simulink model "Color_recog_drone"  (R2023b)
settings: Solver=FixedStepAuto  StartTime=0.0  StopTime=inf  RelTol=1e-3  EnableMultiTasking=on
InitFcn:
  | load('BusDefinitions.mat')
  | codertarget.parrot.internal.checkImageBlocks(gcs)
undefined symbols (not defined in the file): codertarget, gray, Ts
libraries: matrix_library x3, simulink x1, parrotlib x1
settings Model: SimulationMode=external  ExtModeTrigDuration=80  Creator=Thaarun  LastModifiedBy=Thaarun
settings SolverCC: AlgebraicLoopSolver=TrustRegion  PositivePriorityOrder=on
settings OptimizationCC: ReuseModelBlockBuffer=off  PassReuseOutputArgsThreshold=0  MaxStackSize=64
settings DebuggingCC: ParameterTunabilityLossMsg=error  UnconnectedInputMsg=warning  UnconnectedOutputMsg=warning  UnconnectedLineMsg=warning  ArithmeticOperatorsInVariantConditions=warning
settings HardwareCC: ProdBitPerPointer=32  ProdBitPerSizeT=32  ProdBitPerPtrDiffT=32  ProdLargestAtomicInteger=Long  ProdWordSize=32  ProdHWDeviceType=ARM Compatible->ARM 9  UseEmbeddedCoderFeatures=off  UseSimulinkCoderFeatures=off
settings ModelReferenceCC: EnableRefExpFcnMdlSchedulingChecks=on
settings SFSimCC: SimUseLocalCustomCode=off  MATLABDynamicMemAlloc=off
settings RTWCC: Description=Embedded Coder  SystemTargetFile=ert.tlc  HardwareBoard=PARROT Mambo  TemplateMakefile=ert_default_tmf  RTWVerbose=off  RTWUseLocalCustomCode=off  Toolchain=Sourcery G++ Lite GNU Toolchain for Drones  DLArmComputeVersion=19.05
settings CodeAppCC: ForceParamTrailComments=on  OperatorAnnotations=on  MangleLength=10  StateflowObjectComments=on
settings ERTTargetCC: ERTCustomFileBanners=off  SupportContinuousTime=on  SupportNonInlinedSFcns=on  RemoveResetFunc=off  ModelStepFunctionPrototypeControlCompliant=off  ExtMode=on  ExtModeMaxTrigDuration=80  ExtModeMexArgs='192.168.3.1' 1 17725  ERTSrcFileBannerTemplate=codertarget_code_template.cgt  ERTHdrFileBannerTemplate=codertarget_code_template.cgt  ERTDataSrcFileTemplate=codertarget_code_template.cgt  ERTDataHdrFileTemplate=codertarget_code_template.cgt

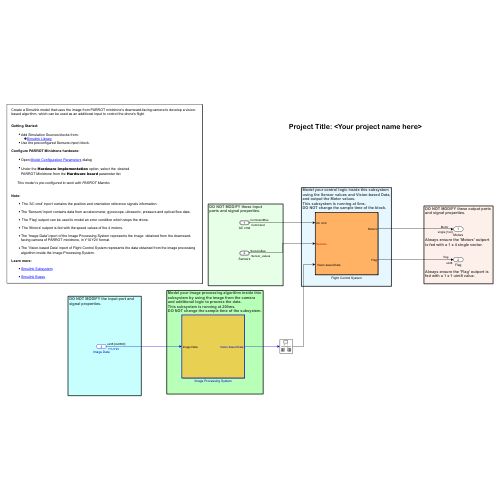
[thumbnail: Simulink's stored preview of the top-level diagram]
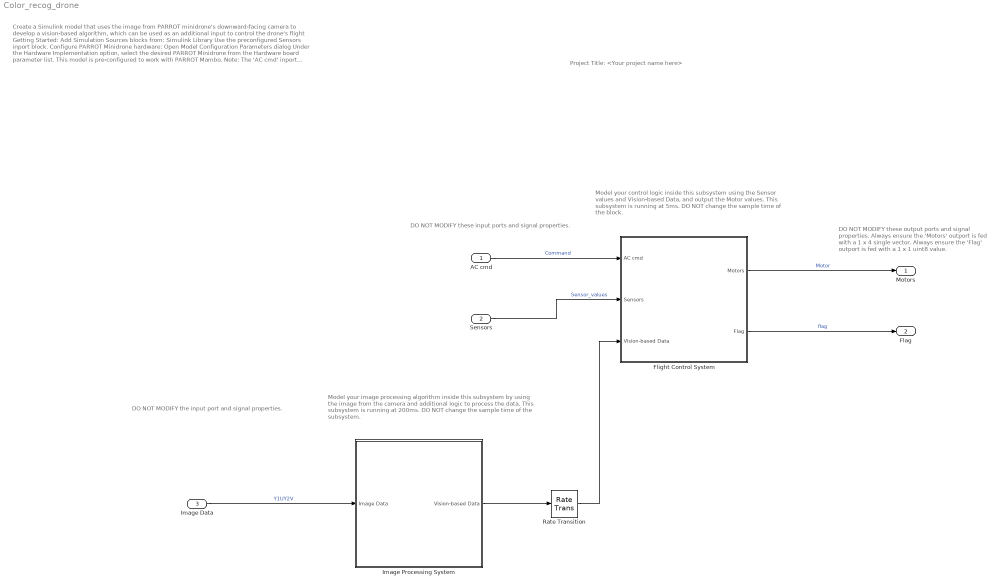
== system Color_recog_drone ==
  note: Model your control logic inside this subsystem
      | using the Sensor values and Vision-based Data,
      | and output the Motor values.
      | This subsystem is running at 5ms.
      | DO NOT change the sample time of the block.
  note: DO NOT MODIFY these output ports
      | and signal properties.
      |
      |
      |
      |
      |
      | Always ensure the 'Motors' outport
      | is fed with a 1 x 4 single vector.
      |
      |
      |
      |
      |
      | Always ensure the 'Flag' outport is
      | fed with a 1 x 1 uint8 value.
  note: DO NOT MODIFY these input
      | ports and signal properties.
  note: Create a Simulink model that uses the image from PARROT minidrone's downward-facing camera to develop a vision-based algorithm, which can be used as an additional input to control the drone's flight
      |
      | Getting Started:
      |
      | Add Simulation Sources blocks from:
      | Simulink Library
      | Use the preconfigured Sensors inport block.
      |
      | Configure PARROT Minidrone hardware:
      |
      | Open Model Configuration Parameters dialog
      |
      | Under the Hardware Implementation option, select the desired
      | PARROT Minidrone from the Hardware board parameter list.
      |
      | This model is pre-configured to work with PARROT Mambo.
      |
      | Note:
      |
      | The 'AC cmd' inport contains the position and orientation reference signals information.
      | The 'Sensors' inport contains data from accelerometer, gyroscope, ultrasonic, pressure and optical flow data.
      | The 'Flag' outport can be used to model an error condition which stops the drone.
      | The 'Motors' outport is fed with the speed values of the 4 motors.
      | The 'Image Data' inport of the Image Processing System represents the image obtained from the downward-facing camera of PARROT minidrone, in Y1UY2V format.
      | The 'Vision-based Data' inport of Flight Control System represents the data obtained from the image processing algorithm inside the Image Processing System.
      | Learn more:
      |
      | Simulink Subsystem
      | Simulink Buses
  note: Project Title: <Your project name here>
  note: DO NOT MODIFY the input port and
      | signal properties.
  note: Model your image processing algorithm inside this
      | subsystem by using the image from the camera
      | and additional logic to process the data.
      | This subsystem is running at 200ms.
      | DO NOT change the sample time of the subsystem.
  AC cmd : Inport  OutDataTypeStr=Bus: CommandBus  BusOutputAsStruct=on
  Sensors : Inport  Port=2  OutDataTypeStr=Bus: SensorsBus  BusOutputAsStruct=on
  Image Data : Inport  Tag=IP_IN  InitFcn=codertarget.parrot.internal.inportCallback(gcb);  Port=3  OutDataTypeStr=uint8  PortDimensions=[4 9600]  BusOutputAsStruct=on
  Flight Control System : Subsystem  InitFcn=codertarget.parrot.internal.fcsSubsystemCallback(gcb);  TreatAsAtomicUnit=on  SystemSampleTime=Ts
  Image Processing System : Subsystem  Tag=IP_SUB  InitFcn=codertarget.parrot.internal.ipSubsystemCallback(gcb);  TreatAsAtomicUnit=on  SystemSampleTime=40*Ts  RTWFcnName=ImageFunction
      settings: RTWSystemCode=Inline  RTWFcnNameOpts=User specified
  Rate Transition : RateTransition  Deterministic=off
  Motors : Outport  OutDataTypeStr=single  PortDimensions=[1 4]  VectorParamsAs1DForOutWhenUnconnected=off
  Flag : Outport  Port=2  OutDataTypeStr=uint8  PortDimensions=1  VectorParamsAs1DForOutWhenUnconnected=off
  wires:
  Flight Control System/1(Motors) -> Motors/1  "Motor"
  AC cmd/1 -> Flight Control System/1(AC cmd)  "Command"
  Sensors/1 -> Flight Control System/2(Sensors)  "Sensor_values"
  Flight Control System/2(Flag) -> Flag/1  "flag"
  Image Data/1 -> Image Processing System/1(Image Data)  "Y1UY2V"
  Rate Transition/1 -> Flight Control System/3(" Vision-based Data")
  Image Processing System/1(" Vision-based Data") -> Rate Transition/1

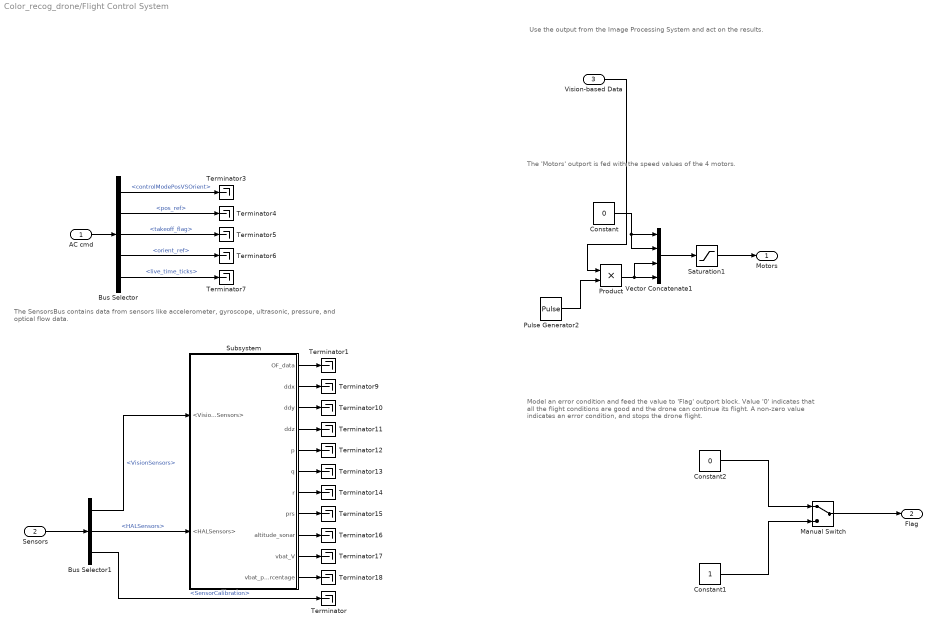
== system Color_recog_drone/Flight Control System ==
  note: The 'Motors' outport is fed with the speed values of the 4 motors.
  note: Model an error condition and feed the value to 'Flag' outport block.
      | Value '0' indicates that all the flight conditions are good and the drone
      | can continue its flight.
      | A non-zero value indicates an error condition, and stops the drone
      | flight.
  note: The SensorsBus contains data from sensors like
      | accelerometer, gyroscope, ultrasonic, pressure,
      | and optical flow data.
  note: Use the output from the Image Processing System and act on the
      | results.
  AC cmd : Inport
  Sensors : Inport  Port=2
  " Vision-based Data" : Inport  Port=3
  Bus Selector : BusSelector  OutputSignals=controlModePosVSOrient,pos_ref,takeoff_flag,orient_ref,live_time_ticks
  Bus Selector1 : BusSelector  OutputSignals=VisionSensors,HALSensors,SensorCalibration
  Constant : Constant  Value=0
  Constant1 : Constant  OutDataTypeStr=uint8
  Constant2 : Constant  Value=0  OutDataTypeStr=uint8
  Manual Switch : ManualSwitch
  Product : Product
  Pulse Generator2 : DiscretePulseGenerator  Amplitude=400  Period=800  PulseWidth=400  PhaseDelay=400  SampleTime=Ts
  Saturation1 : Saturate  UpperLimit=500  LowerLimit=0  OutDataTypeStr=single
  Subsystem : Subsystem
  Terminator{,1,3..7,9..18} (17 alike) : Terminator
  Vector Concatenate1 : Concatenate  NumInputs=4
  Motors : Outport  VectorParamsAs1DForOutWhenUnconnected=off
  Flag : Outport  Port=2  VectorParamsAs1DForOutWhenUnconnected=off
  wires:
  AC cmd/1 -> Bus Selector/1
  Sensors/1 -> Bus Selector1/1
  Bus Selector/1 -> Terminator3/1  "<controlModePosVSOrient>"
  Bus Selector/2 -> Terminator4/1  "<pos_ref>"
  Bus Selector/3 -> Terminator5/1  "<takeoff_flag>"
  Bus Selector/4 -> Terminator6/1  "<orient_ref>"
  Bus Selector/5 -> Terminator7/1  "<live_time_ticks>"
  Manual Switch/1 -> Flag/1
  Constant2/1 -> Manual Switch/1
  Constant1/1 -> Manual Switch/2
  Vector Concatenate1/1 -> Saturation1/1
  Pulse Generator2/1 -> Product/2
  Saturation1/1 -> Motors/1
  Bus Selector1/1 -> Subsystem/1(<VisionSensors>)  "<VisionSensors>"
  Bus Selector1/2 -> Subsystem/2(<HALSensors>)  "<HALSensors>"
  Bus Selector1/3 -> Terminator/1  "<SensorCalibration>"
  Subsystem/1(OF_data) -> Terminator1/1
  Subsystem/2(ddx) -> Terminator9/1
  Subsystem/3(ddy) -> Terminator10/1
  Subsystem/4(ddz) -> Terminator11/1
  Subsystem/5(p) -> Terminator12/1
  Subsystem/7(r) -> Terminator14/1
  Subsystem/8(prs) -> Terminator15/1
  Subsystem/9(altitude_sonar) -> Terminator16/1
  Subsystem/10(vbat_V) -> Terminator17/1
  Subsystem/11(vbat_percentage) -> Terminator18/1
  Subsystem/6(q) -> Terminator13/1
  Constant/1 -> Vector Concatenate1/2, Vector Concatenate1/1
  " Vision-based Data"/1 -> Product/1
  Product/1 -> Vector Concatenate1/3, Vector Concatenate1/4

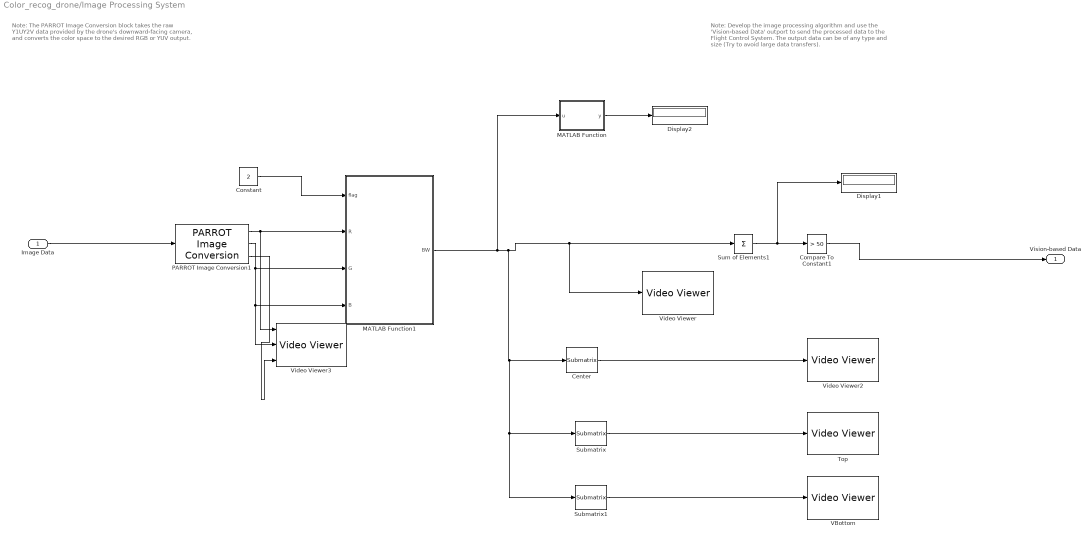
== system Color_recog_drone/Image Processing System ==
  note: Note:
      |
      | Develop the image processing algorithm and use the 'Vision-based Data' outport to send the processed data to the Flight Control System. The output data can be of any type and size (Try to avoid large data transfers).
  note: Note:
      |
      | The PARROT Image Conversion block takes the raw Y1UY2V data provided by the drone's downward-facing camera, and converts the color space to the desired RGB or YUV output.
  Image Data : Inport
  Center : matrix_library/Submatrix  RowSpan=Range of rows  RowStartMode=Offset from middle  RowStartIndex=-10  RowEndMode=Offset from middle  RowEndIndex=10  ColSpan=Range of columns  ColStartMode=Offset from middle  ColStartIndex=-10  ColEndMode=Offset from middle  ColEndIndex=10
  Compare To Constant1 : simulink/Logic and Bit Operations/Compare To Constant  relop=>  const=50  OutDataTypeStr=boolean
  Constant : Constant  Value=2  OutDataTypeStr=int8
  Display1 : Display
  Display2 : Display
  MATLAB Function : MATLAB Function  TreatAsAtomicUnit=on
  MATLAB Function1 : MATLAB Function  TreatAsAtomicUnit=on
  PARROT Image Conversion1 : parrotlib/PARROT Image Conversion  Tag=IP_FORMAT  ImageFormat=RGB  R=on  Y=on  G=on  U=on  B=on  V=on
  Submatrix : matrix_library/Submatrix  RowSpan=Range of rows  RowStartMode=First  RowStartIndex=10  RowEndMode=Index  RowEndIndex=30  ColSpan=Range of columns  ColStartMode=First  ColStartIndex=-10  ColEndMode=Last  ColEndIndex=10
  Submatrix1 : matrix_library/Submatrix  RowSpan=Range of rows  RowStartMode=Index  RowStartIndex=90  RowEndMode=Last  RowEndIndex=30  ColSpan=Range of columns  ColStartMode=First  ColStartIndex=-10  ColEndMode=Last  ColEndIndex=10
  Sum of Elements1 : Sum  Inputs=+  OutDataTypeStr=uint16
  Top : VideoViewer  colormapValue=gray(256)  FigPos=[957 1001.2 417.6 304]
  VBottom : VideoViewer  colormapValue=gray(256)  FigPos=[29.8 702 417.6 304]
  Video Viewer : VideoViewer  colormapValue=gray(256)  FigPos=[969 641.2 424.8 352.8]
  Video Viewer2 : VideoViewer  colormapValue=gray(256)  FigPos=[1096.2 1246.8 567.2 484]
  Video Viewer3 : VideoViewer  imagePorts=separate color signals  colormapValue=gray(256)  FigPos=[122.6 846.8 766.4 672]
  " Vision-based Data" : Outport  VectorParamsAs1DForOutWhenUnconnected=off
  wires:
  PARROT Image Conversion1/1 -> Video Viewer3/1, MATLAB Function1/2(R)
  MATLAB Function1/1(BW) -> MATLAB Function/1(u), Submatrix1/1, Submatrix/1, Center/1, Video Viewer/1, Sum of Elements1/1
  PARROT Image Conversion1/2 -> Video Viewer3/2, MATLAB Function1/4(B), MATLAB Function1/3(G)
  Sum of Elements1/1 -> Display1/1, Compare To Constant1/1
  Image Data/1 -> PARROT Image Conversion1/1
  PARROT Image Conversion1/3 -> Video Viewer3/3
  Compare To Constant1/1 -> " Vision-based Data"/1
  MATLAB Function/1(y) -> Display2/1
  Center/1 -> Video Viewer2/1
  Submatrix/1 -> Top/1
  Submatrix1/1 -> VBottom/1
  Constant/1 -> MATLAB Function1/1(flag)

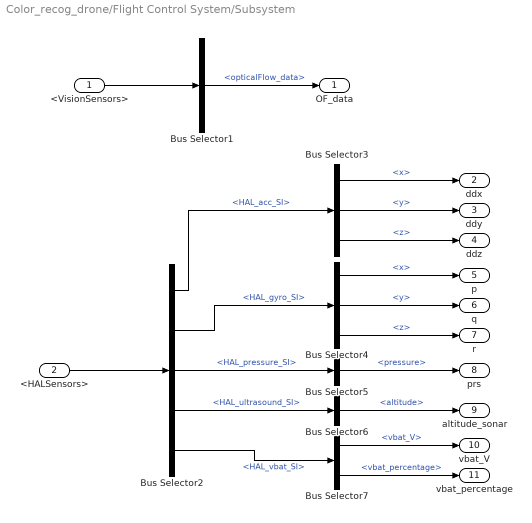
== system Color_recog_drone/Flight Control System/Subsystem ==
  <VisionSensors> : Inport
  <HALSensors> : Inport  Port=2
  Bus Selector1 : BusSelector  OutputSignals=opticalFlow_data
  Bus Selector2 : BusSelector  OutputSignals=HAL_acc_SI,HAL_gyro_SI,HAL_pressure_SI,HAL_ultrasound_SI,HAL_vbat_SI
  Bus Selector3 : BusSelector  OutputSignals=x,y,z
  Bus Selector4 : BusSelector  OutputSignals=x,y,z
  Bus Selector5 : BusSelector  OutputSignals=pressure
  Bus Selector6 : BusSelector  OutputSignals=altitude
  Bus Selector7 : BusSelector  OutputSignals=vbat_V,vbat_percentage
  OF_data : Outport  VectorParamsAs1DForOutWhenUnconnected=off
  ddx : Outport  Port=2  VectorParamsAs1DForOutWhenUnconnected=off
  ddy : Outport  Port=3  VectorParamsAs1DForOutWhenUnconnected=off
  ddz : Outport  Port=4  VectorParamsAs1DForOutWhenUnconnected=off
  p : Outport  Port=5  VectorParamsAs1DForOutWhenUnconnected=off
  q : Outport  Port=6  VectorParamsAs1DForOutWhenUnconnected=off
  r : Outport  Port=7  VectorParamsAs1DForOutWhenUnconnected=off
  prs : Outport  Port=8  VectorParamsAs1DForOutWhenUnconnected=off
  altitude_sonar : Outport  Port=9  VectorParamsAs1DForOutWhenUnconnected=off
  vbat_V : Outport  Port=10  VectorParamsAs1DForOutWhenUnconnected=off
  vbat_percentage : Outport  Port=11  VectorParamsAs1DForOutWhenUnconnected=off
  wires:
  <VisionSensors>/1 -> Bus Selector1/1
  <HALSensors>/1 -> Bus Selector2/1
  Bus Selector1/1 -> OF_data/1  "<opticalFlow_data>"
  Bus Selector2/1 -> Bus Selector3/1  "<HAL_acc_SI>"
  Bus Selector2/2 -> Bus Selector4/1  "<HAL_gyro_SI>"
  Bus Selector2/3 -> Bus Selector5/1  "<HAL_pressure_SI>"
  Bus Selector2/4 -> Bus Selector6/1  "<HAL_ultrasound_SI>"
  Bus Selector2/5 -> Bus Selector7/1  "<HAL_vbat_SI>"
  Bus Selector3/1 -> ddx/1  "<x>"
  Bus Selector3/2 -> ddy/1  "<y>"
  Bus Selector3/3 -> ddz/1  "<z>"
  Bus Selector4/2 -> q/1  "<y>"
  Bus Selector4/1 -> p/1  "<x>"
  Bus Selector4/3 -> r/1  "<z>"
  Bus Selector5/1 -> prs/1  "<pressure>"
  Bus Selector6/1 -> altitude_sonar/1  "<altitude>"
  Bus Selector7/1 -> vbat_V/1  "<vbat_V>"
  Bus Selector7/2 -> vbat_percentage/1  "<vbat_percentage>"

== matlab function Color_recog_drone/Image Processing System/MATLAB Function1 ==
  data: flag input; R input; BW output; G input; B input
function BW  = createMask(flag,R,G,B)
%createMask  Threshold RGB image using auto-generated code from colorThresholder app.
%  [BW,MASKEDRGBIMAGE] = createMask(RGB) thresholds image RGB using
%  auto-generated code from the colorThresholder app. The colorspace and
%  range for each channel of the colorspace were set within the app. The
%  segmentation mask is returned in BW, and a composite of the mask and
%  original RGB images is returned in maskedRGBImage.

% Auto-generated by colorThresholder app on 03-Feb-2024
%------------------------------------------------------

I = cat(3,R,G,B)
HSV = rgb2hsv(I)
[H,S,V] = imsplit(HSV)

% Convert RGB image to chosen color space

if flag == 1
% Define thresholds for channel 1 based on histogram settings
channel1Min = 222.000;
channel1Max = 255.000;

% Define thresholds for channel 2 based on histogram settings
channel2Min = 113.000;
channel2Max = 223.000;

% Define thresholds for channel 3 based on histogram settings
channel3Min = 132.000;
channel3Max = 242.000;




% Create mask based on chosen histogram thresholds
sliderBW = (R >= channel1Min ) & (R <= channel1Max) & ...
    (G >= channel2Min ) & (G <= channel2Max) & ...
    (B >= channel3Min ) & (B <= channel3Max);
BW = sliderBW;


elseif flag ==2
% Define thresholds for channel 1 based on histogram settings
channel1Min = 0.894;
channel1Max = 0.002;

% Define thresholds for channel 2 based on histogram settings
channel2Min = 0.180;
channel2Max = 0.628;

% Define thresholds for channel 3 based on histogram settings
channel3Min = 0.463;
channel3Max = 1.000;



sliderBW = ( H >= channel1Min) | (H <= channel1Max)  & ...
    (S >= channel2Min ) & (S <= channel2Max) & ...
    (V >= channel3Min ) & (V <= channel3Max);

% Create mask based on chosen histogram thresholds

BW = sliderBW;
elseif flag == 3
% Define thresholds for channel 1 based on histogram settings
channel1Min = 0.563;
channel1Max = 0.719;

% Define thresholds for channel 2 based on histogram settings
channel2Min = 0.307;
channel2Max = 1.000;

% Define thresholds for channel 3 based on histogram settings
channel3Min = 0.396;
channel3Max = 1.000;




% Create mask based on chosen histogram thresholds
sliderBW = (H >= channel1Min ) & (H <= channel1Max) & ...
    (S >= channel2Min ) & (S <= channel2Max) & ...
    (V >= channel3Min ) & (V <= channel3Max);
BW = sliderBW;
elseif flag == 4
% Define thresholds for channel 1 based on histogram settings
channel1Min = 0.118;
channel1Max = 0.183;

% Define thresholds for channel 2 based on histogram settings
channel2Min = 0.122;
channel2Max = 1.000;

% Define thresholds for channel 3 based on histogram settings
channel3Min = 0.852;
channel3Max = 1.000;





% Create mask based on chosen histogram thresholds
sliderBW = (H >= channel1Min ) & (H <= channel1Max) & ...
    (S >= channel2Min ) & (S <= channel2Max) & ...
    (V >= channel3Min ) & (V <= channel3Max);
BW = sliderBW;
else
       % Define thresholds for channel 1 based on histogram settings
channel1Min = 236.000;
channel1Max = 255.000;

% Define thresholds for channel 2 based on histogram settings
channel2Min = 0.000;
channel2Max = 255.000;

% Define thresholds for channel 3 based on histogram settings
channel3Min = 0.000;
channel3Max = 255.000;


% Create mask based on chosen histogram thresholds
sliderBW = (R >= channel1Min ) & (R <= channel1Max) & ...
    (G >= channel2Min ) & (G <= channel2Max) & ...
    (B >= channel3Min ) & (B <= channel3Max);
BW = sliderBW;
    BW = sliderBW
end

end

== matlab function Color_recog_drone/Image Processing System/MATLAB Function ==
  data: u input; y output
function y = fcn(u)

y = u(100,100);
